simulink model "pfb_core_snbxfft32"  (R2012b)
settings: Solver=FixedStepDiscrete  SolverMode=SingleTasking  StartTime=0.0  StopTime=5000  FixedStep=1  RelTol=1e-3
undefined symbols (not defined in the file or in its folder): xlipgetpartsetting
undefined symbols (not defined in the file): pfb_coeff_gen_calc
libraries: xbsIndex_r4 x5100, casper_library_misc x2, casper_library_delays x1
(part 4 of 18)

== system pfb_core_snbxfft32/pfb/pfb_fir_generic/pfb_fir_coeff_gen/rom ==
  addra : Inport
  dina : Inport  Port=2
  wea : Inport  Port=3
  addrb : Inport  Port=4
  dinb : Inport  Port=5
  web : Inport  Port=6
  A_bussify : Subsystem  AncestorBlock=casper_library_flow_control/bus_create  mask(bus_create){inputNum=72}
      mask prompts: inputNum "Number of inputs:"
      mask init:
      | bus_create_init(gcb,...
      |     'inputNum', inputNum);
  B_bussify : Subsystem  AncestorBlock=casper_library_flow_control/bus_create  mask(bus_create){inputNum=72}
      mask prompts: inputNum "Number of inputs:"
      mask init:
      | bus_create_init(gcb,...
      |     'inputNum', inputNum);
  bram{0..71} (72 alike) : xbsIndex_r4/Dual Port RAM  depth=65536  initVector=getfield(get_param(gcb, 'UserData'), 'initVector')  distributed_mem=Block RAM  init_a=0  init_b=0  rst_a=off  rst_b=off  en_a=off  en_b=off  latency=8  write_mode_A=Read Before Write  write_mode_B=Read Before Write  dbl_ovrd=off  optimize=Speed  block_type=dpram
  ddina : xbsIndex_r4/Delay  rst=off  infoeditControl=Selection of Reset will increase slice count due to use of real FFs and instead of SRLs  en=off  latency=0  dbl_ovrd=off  reg_retiming=on  block_type=delay
  ddinb : xbsIndex_r4/Delay  rst=off  infoeditControl=Selection of Reset will increase slice count due to use of real FFs and instead of SRLs  en=off  latency=0  dbl_ovrd=off  reg_retiming=on  block_type=delay
  debus_addra : Subsystem  AncestorBlock=casper_library_flow_control/bus_expand  mask(bus_expand){mode=divisions of equal size, outputNum=72, outputWidth=[16 16 16 16 16 16 16 16 16 16 16 16 16 16 16 16 16 16 16 16 16 16 16 16 16 16 16 16 16 16 16 16 16 16 16 16 16 16 16 16 16 16 16 16 16 16 16 16 16 16 16 16 16 16 16 16 16 16 16 16 16 16 16 16 16 16 16 16 16 16 16 16], outputBinaryPt=[0 0 0 0 0 0 0 0 0 0 0 0 0 0 0 0 0 0 0 0 0 0 0 0 0 0 0 0 0 0 0 0 0 0 0 0 0 0 0 0 0 0 0 0 0 0 0 0 0 0 0 0 0 0 0 0 0 0 0 0 0 0 0 0 0 0 0 0 0 0 0 0], outputArithmeticType=[0 0 0 0 0 0 0 0 0 0 0 0 0 0 0 0 0 0 0 0 0 0 0 0 0 0 0 0 0 0 0 0 0 0 0 0 0 0 0 0 0 0 0 0 0 0 0 0 0 0 0 0 0 0 0 0 0 0 0 0 0 0 0 0 0 0 0 0 0 0 0 0], show_format=on, outputToWorkspace=off, variablePrefix=, outputToModelAsWell=on}
      mask prompts: outputNum "Number of outputs:"; outputWidth "Output width:"; outputBinaryPt "Output binary point position:"; outputArithmeticType "Output arithmetic type (ufix=0, fix=1, bool=2):"; show_format "Print format string?"; outputToWorkspace "Output to workspace?"; variablePrefix "Variable name prefix:"; outputToModelAsWell "Output to model as well?"
      mask help:
      | Expands a 'bus' made using a bus_create or Xilinx
      | concat block.
      | The input will be divided into the specified number
      | of outputs with the specified arithmetic types.
      | Divisions are made from most significant bit.
      mask init: same as pfb_core_snbxfft32/pfb/pfb_fir_generic/bus_expand
      settings: AttributesFormatString=72 outputs: uf16.0,uf16.0,uf16.0,uf16.0,uf16.0,uf16.0,uf16.0,uf16.0,uf16.0,uf16.0,uf16.0,uf16.0,uf16.0,uf16.0,uf16.0,uf16.0,uf16.0,uf16.0,uf16.0,uf16.0,uf16.0,uf16.0,uf16.0,uf16.0,uf16.0,uf16.0,uf16.0,uf16.0,uf16.0,uf16.0,uf16.0,uf16.0,uf16.0,uf16.0,uf16.0,uf16.0,uf16.0,uf16.0,uf16.0,uf16.0,uf16.0,uf16.0,uf16.0,uf16.0,uf16.0,uf16.0,uf16.0,uf16.0,uf16.0,uf16.0,uf16.0,uf16.0,uf16.0,uf16.0,uf16.0,uf16.0,uf16.0,uf16.0,uf16.0,uf16.0,uf16.0,uf16.0,uf16.0,uf16.0,uf16.0,uf16.0,uf16.0,uf16.0,uf16.0,uf16.0,uf16.0,uf16.0,
      mask TypeOptions mode: divisions of equal size | divisions of arbitrary size
      mask Callback mode: bus_expand_callback();
      mask Callback outputWidth: bus_expand_callback();
      mask Callback outputToWorkspace: bus_expand_callback();
  debus_addrb : Subsystem  AncestorBlock=casper_library_flow_control/bus_expand  mask(bus_expand){mode=divisions of equal size, outputNum=72, outputWidth=[16 16 16 16 16 16 16 16 16 16 16 16 16 16 16 16 16 16 16 16 16 16 16 16 16 16 16 16 16 16 16 16 16 16 16 16 16 16 16 16 16 16 16 16 16 16 16 16 16 16 16 16 16 16 16 16 16 16 16 16 16 16 16 16 16 16 16 16 16 16 16 16], outputBinaryPt=[0 0 0 0 0 0 0 0 0 0 0 0 0 0 0 0 0 0 0 0 0 0 0 0 0 0 0 0 0 0 0 0 0 0 0 0 0 0 0 0 0 0 0 0 0 0 0 0 0 0 0 0 0 0 0 0 0 0 0 0 0 0 0 0 0 0 0 0 0 0 0 0], outputArithmeticType=[0 0 0 0 0 0 0 0 0 0 0 0 0 0 0 0 0 0 0 0 0 0 0 0 0 0 0 0 0 0 0 0 0 0 0 0 0 0 0 0 0 0 0 0 0 0 0 0 0 0 0 0 0 0 0 0 0 0 0 0 0 0 0 0 0 0 0 0 0 0 0 0], show_format=on, outputToWorkspace=off, variablePrefix=, outputToModelAsWell=on}
      mask prompts: outputNum "Number of outputs:"; outputWidth "Output width:"; outputBinaryPt "Output binary point position:"; outputArithmeticType "Output arithmetic type (ufix=0, fix=1, bool=2):"; show_format "Print format string?"; outputToWorkspace "Output to workspace?"; variablePrefix "Variable name prefix:"; outputToModelAsWell "Output to model as well?"
      mask help:
      | Expands a 'bus' made using a bus_create or Xilinx
      | concat block.
      | The input will be divided into the specified number
      | of outputs with the specified arithmetic types.
      | Divisions are made from most significant bit.
      mask init: same as pfb_core_snbxfft32/pfb/pfb_fir_generic/bus_expand
      settings: AttributesFormatString=72 outputs: uf16.0,uf16.0,uf16.0,uf16.0,uf16.0,uf16.0,uf16.0,uf16.0,uf16.0,uf16.0,uf16.0,uf16.0,uf16.0,uf16.0,uf16.0,uf16.0,uf16.0,uf16.0,uf16.0,uf16.0,uf16.0,uf16.0,uf16.0,uf16.0,uf16.0,uf16.0,uf16.0,uf16.0,uf16.0,uf16.0,uf16.0,uf16.0,uf16.0,uf16.0,uf16.0,uf16.0,uf16.0,uf16.0,uf16.0,uf16.0,uf16.0,uf16.0,uf16.0,uf16.0,uf16.0,uf16.0,uf16.0,uf16.0,uf16.0,uf16.0,uf16.0,uf16.0,uf16.0,uf16.0,uf16.0,uf16.0,uf16.0,uf16.0,uf16.0,uf16.0,uf16.0,uf16.0,uf16.0,uf16.0,uf16.0,uf16.0,uf16.0,uf16.0,uf16.0,uf16.0,uf16.0,uf16.0,
      mask TypeOptions mode: divisions of equal size | divisions of arbitrary size
      mask Callback mode: bus_expand_callback();
      mask Callback outputWidth: bus_expand_callback();
      mask Callback outputToWorkspace: bus_expand_callback();
  debus_dina : Subsystem  AncestorBlock=casper_library_flow_control/bus_expand  mask(bus_expand){mode=divisions of arbitrary size, outputNum=1, outputWidth=[1 1 1 1 1 1 1 1 1 1 1 1 1 1 1 1 1 1 1 1 1 1 1 1 1 1 1 1 1 1 1 1 1 1 1 1 1 1 1 1 1 1 1 1 1 1 1 1 1 1 1 1 1 1 1 1 1 1 1 1 1 1 1 1 1 1 1 1 1 1 1 1], outputBinaryPt=[0 0 0 0 0 0 0 0 0 0 0 0 0 0 0 0 0 0 0 0 0 0 0 0 0 0 0 0 0 0 0 0 0 0 0 0 0 0 0 0 0 0 0 0 0 0 0 0 0 0 0 0 0 0 0 0 0 0 0 0 0 0 0 0 0 0 0 0 0 0 0 0], outputArithmeticType=[0 0 0 0 0 0 0 0 0 0 0 0 0 0 0 0 0 0 0 0 0 0 0 0 0 0 0 0 0 0 0 0 0 0 0 0 0 0 0 0 0 0 0 0 0 0 0 0 0 0 0 0 0 0 0 0 0 0 0 0 0 0 0 0 0 0 0 0 0 0 0 0], show_format=on, outputToWorkspace=off, variablePrefix=, outputToModelAsWell=on}
      mask prompts: outputNum "Number of outputs:"; outputWidth "Output width [msb ... lsb]:"; outputBinaryPt "Output binary point position [msb ... lsb]:"; outputArithmeticType "Output arithmetic type (ufix=0, fix=1, bool=2) [msb ... lsb]:"; show_format "Print format string?"; outputToWorkspace "Output to workspace?"; variablePrefix "Variable name prefix:"; outputToModelAsWell "Output to model as well?"
      mask help:
      | Expands a 'bus' made using a bus_create or Xilinx
      | concat block.
      | The input will be divided into the specified number
      | of outputs with the specified arithmetic types.
      | Divisions are made from most significant bit.
      mask init: same as pfb_core_snbxfft32/pfb/pfb_fir_generic/bus_expand
      settings: AttributesFormatString=72 outputs: uf1.0,uf1.0,uf1.0,uf1.0,uf1.0,uf1.0,uf1.0,uf1.0,uf1.0,uf1.0,uf1.0,uf1.0,uf1.0,uf1.0,uf1.0,uf1.0,uf1.0,uf1.0,uf1.0,uf1.0,uf1.0,uf1.0,uf1.0,uf1.0,uf1.0,uf1.0,uf1.0,uf1.0,uf1.0,uf1.0,uf1.0,uf1.0,uf1.0,uf1.0,uf1.0,uf1.0,uf1.0,uf1.0,uf1.0,uf1.0,uf1.0,uf1.0,uf1.0,uf1.0,uf1.0,uf1.0,uf1.0,uf1.0,uf1.0,uf1.0,uf1.0,uf1.0,uf1.0,uf1.0,uf1.0,uf1.0,uf1.0,uf1.0,uf1.0,uf1.0,uf1.0,uf1.0,uf1.0,uf1.0,uf1.0,uf1.0,uf1.0,uf1.0,uf1.0,uf1.0,uf1.0,uf1.0,
      mask TypeOptions mode: divisions of equal size | divisions of arbitrary size
      mask Callback mode: bus_expand_callback();
      mask Callback outputWidth: bus_expand_callback();
      mask Callback outputToWorkspace: bus_expand_callback();
  debus_dinb : Subsystem  AncestorBlock=casper_library_flow_control/bus_expand  mask(bus_expand){mode=divisions of arbitrary size, outputNum=1, outputWidth=[1 1 1 1 1 1 1 1 1 1 1 1 1 1 1 1 1 1 1 1 1 1 1 1 1 1 1 1 1 1 1 1 1 1 1 1 1 1 1 1 1 1 1 1 1 1 1 1 1 1 1 1 1 1 1 1 1 1 1 1 1 1 1 1 1 1 1 1 1 1 1 1], outputBinaryPt=[0 0 0 0 0 0 0 0 0 0 0 0 0 0 0 0 0 0 0 0 0 0 0 0 0 0 0 0 0 0 0 0 0 0 0 0 0 0 0 0 0 0 0 0 0 0 0 0 0 0 0 0 0 0 0 0 0 0 0 0 0 0 0 0 0 0 0 0 0 0 0 0], outputArithmeticType=[0 0 0 0 0 0 0 0 0 0 0 0 0 0 0 0 0 0 0 0 0 0 0 0 0 0 0 0 0 0 0 0 0 0 0 0 0 0 0 0 0 0 0 0 0 0 0 0 0 0 0 0 0 0 0 0 0 0 0 0 0 0 0 0 0 0 0 0 0 0 0 0], show_format=on, outputToWorkspace=off, variablePrefix=, outputToModelAsWell=on}
      mask prompts: outputNum "Number of outputs:"; outputWidth "Output width [msb ... lsb]:"; outputBinaryPt "Output binary point position [msb ... lsb]:"; outputArithmeticType "Output arithmetic type (ufix=0, fix=1, bool=2) [msb ... lsb]:"; show_format "Print format string?"; outputToWorkspace "Output to workspace?"; variablePrefix "Variable name prefix:"; outputToModelAsWell "Output to model as well?"
      mask help:
      | Expands a 'bus' made using a bus_create or Xilinx
      | concat block.
      | The input will be divided into the specified number
      | of outputs with the specified arithmetic types.
      | Divisions are made from most significant bit.
      mask init: same as pfb_core_snbxfft32/pfb/pfb_fir_generic/bus_expand
      settings: AttributesFormatString=72 outputs: uf1.0,uf1.0,uf1.0,uf1.0,uf1.0,uf1.0,uf1.0,uf1.0,uf1.0,uf1.0,uf1.0,uf1.0,uf1.0,uf1.0,uf1.0,uf1.0,uf1.0,uf1.0,uf1.0,uf1.0,uf1.0,uf1.0,uf1.0,uf1.0,uf1.0,uf1.0,uf1.0,uf1.0,uf1.0,uf1.0,uf1.0,uf1.0,uf1.0,uf1.0,uf1.0,uf1.0,uf1.0,uf1.0,uf1.0,uf1.0,uf1.0,uf1.0,uf1.0,uf1.0,uf1.0,uf1.0,uf1.0,uf1.0,uf1.0,uf1.0,uf1.0,uf1.0,uf1.0,uf1.0,uf1.0,uf1.0,uf1.0,uf1.0,uf1.0,uf1.0,uf1.0,uf1.0,uf1.0,uf1.0,uf1.0,uf1.0,uf1.0,uf1.0,uf1.0,uf1.0,uf1.0,uf1.0,
      mask TypeOptions mode: divisions of equal size | divisions of arbitrary size
      mask Callback mode: bus_expand_callback();
      mask Callback outputWidth: bus_expand_callback();
      mask Callback outputToWorkspace: bus_expand_callback();
  debus_wea : Subsystem  AncestorBlock=casper_library_flow_control/bus_expand  mask(bus_expand){mode=divisions of equal size, outputNum=72, outputWidth=[1 1 1 1 1 1 1 1 1 1 1 1 1 1 1 1 1 1 1 1 1 1 1 1 1 1 1 1 1 1 1 1 1 1 1 1 1 1 1 1 1 1 1 1 1 1 1 1 1 1 1 1 1 1 1 1 1 1 1 1 1 1 1 1 1 1 1 1 1 1 1 1], outputBinaryPt=[0 0 0 0 0 0 0 0 0 0 0 0 0 0 0 0 0 0 0 0 0 0 0 0 0 0 0 0 0 0 0 0 0 0 0 0 0 0 0 0 0 0 0 0 0 0 0 0 0 0 0 0 0 0 0 0 0 0 0 0 0 0 0 0 0 0 0 0 0 0 0 0], outputArithmeticType=[2 2 2 2 2 2 2 2 2 2 2 2 2 2 2 2 2 2 2 2 2 2 2 2 2 2 2 2 2 2 2 2 2 2 2 2 2 2 2 2 2 2 2 2 2 2 2 2 2 2 2 2 2 2 2 2 2 2 2 2 2 2 2 2 2 2 2 2 2 2 2 2], show_format=on, outputToWorkspace=off, variablePrefix=, outputToModelAsWell=on}
      mask prompts: outputNum "Number of outputs:"; outputWidth "Output width:"; outputBinaryPt "Output binary point position:"; outputArithmeticType "Output arithmetic type (ufix=0, fix=1, bool=2):"; show_format "Print format string?"; outputToWorkspace "Output to workspace?"; variablePrefix "Variable name prefix:"; outputToModelAsWell "Output to model as well?"
      mask help:
      | Expands a 'bus' made using a bus_create or Xilinx
      | concat block.
      | The input will be divided into the specified number
      | of outputs with the specified arithmetic types.
      | Divisions are made from most significant bit.
      mask init: same as pfb_core_snbxfft32/pfb/pfb_fir_generic/bus_expand
      settings: AttributesFormatString=72 outputs: b,b,b,b,b,b,b,b,b,b,b,b,b,b,b,b,b,b,b,b,b,b,b,b,b,b,b,b,b,b,b,b,b,b,b,b,b,b,b,b,b,b,b,b,b,b,b,b,b,b,b,b,b,b,b,b,b,b,b,b,b,b,b,b,b,b,b,b,b,b,b,b,
      mask TypeOptions mode: divisions of equal size | divisions of arbitrary size
      mask Callback mode: bus_expand_callback();
      mask Callback outputWidth: bus_expand_callback();
      mask Callback outputToWorkspace: bus_expand_callback();
  debus_web : Subsystem  AncestorBlock=casper_library_flow_control/bus_expand  mask(bus_expand){mode=divisions of equal size, outputNum=72, outputWidth=[1 1 1 1 1 1 1 1 1 1 1 1 1 1 1 1 1 1 1 1 1 1 1 1 1 1 1 1 1 1 1 1 1 1 1 1 1 1 1 1 1 1 1 1 1 1 1 1 1 1 1 1 1 1 1 1 1 1 1 1 1 1 1 1 1 1 1 1 1 1 1 1], outputBinaryPt=[0 0 0 0 0 0 0 0 0 0 0 0 0 0 0 0 0 0 0 0 0 0 0 0 0 0 0 0 0 0 0 0 0 0 0 0 0 0 0 0 0 0 0 0 0 0 0 0 0 0 0 0 0 0 0 0 0 0 0 0 0 0 0 0 0 0 0 0 0 0 0 0], outputArithmeticType=[2 2 2 2 2 2 2 2 2 2 2 2 2 2 2 2 2 2 2 2 2 2 2 2 2 2 2 2 2 2 2 2 2 2 2 2 2 2 2 2 2 2 2 2 2 2 2 2 2 2 2 2 2 2 2 2 2 2 2 2 2 2 2 2 2 2 2 2 2 2 2 2], show_format=on, outputToWorkspace=off, variablePrefix=, outputToModelAsWell=on}
      mask prompts: outputNum "Number of outputs:"; outputWidth "Output width:"; outputBinaryPt "Output binary point position:"; outputArithmeticType "Output arithmetic type (ufix=0, fix=1, bool=2):"; show_format "Print format string?"; outputToWorkspace "Output to workspace?"; variablePrefix "Variable name prefix:"; outputToModelAsWell "Output to model as well?"
      mask help:
      | Expands a 'bus' made using a bus_create or Xilinx
      | concat block.
      | The input will be divided into the specified number
      | of outputs with the specified arithmetic types.
      | Divisions are made from most significant bit.
      mask init: same as pfb_core_snbxfft32/pfb/pfb_fir_generic/bus_expand
      settings: AttributesFormatString=72 outputs: b,b,b,b,b,b,b,b,b,b,b,b,b,b,b,b,b,b,b,b,b,b,b,b,b,b,b,b,b,b,b,b,b,b,b,b,b,b,b,b,b,b,b,b,b,b,b,b,b,b,b,b,b,b,b,b,b,b,b,b,b,b,b,b,b,b,b,b,b,b,b,b,
      mask TypeOptions mode: divisions of equal size | divisions of arbitrary size
      mask Callback mode: bus_expand_callback();
      mask Callback outputWidth: bus_expand_callback();
      mask Callback outputToWorkspace: bus_expand_callback();
  rep_addra : Subsystem  AncestorBlock=casper_library_bus/bus_replicate  mask(bus_replicate){replication=72, latency=9, misc=off, implementation=core}
      mask prompts: replication "replication factor"; misc "misc support"; implementation "delay implementation"
      mask help: Output bus formed by replicating input bus a number of times
      mask init:
      | bus_replicate_init(gcb, ...
      |     'replication', replication, ...
      |     'latency', latency, ...
      |     'implementation', implementation, ...
      |     'misc', misc);
      mask TypeOptions implementation: core | behavioral
  rep_addrb : Subsystem  AncestorBlock=casper_library_bus/bus_replicate  mask(bus_replicate){replication=72, latency=9, misc=off, implementation=core}
      mask prompts: replication "replication factor"; misc "misc support"; implementation "delay implementation"
      mask help: Output bus formed by replicating input bus a number of times
      mask init:
      | bus_replicate_init(gcb, ...
      |     'replication', replication, ...
      |     'latency', latency, ...
      |     'implementation', implementation, ...
      |     'misc', misc);
      mask TypeOptions implementation: core | behavioral
  rep_wea : Subsystem  AncestorBlock=casper_library_bus/bus_replicate  mask(bus_replicate){replication=72, latency=0, misc=off, implementation=behavioral}
      mask prompts: replication "replication factor"; misc "misc support"; implementation "delay implementation"
      mask help: Output bus formed by replicating input bus a number of times
      mask init:
      | bus_replicate_init(gcb, ...
      |     'replication', replication, ...
      |     'latency', latency, ...
      |     'implementation', implementation, ...
      |     'misc', misc);
      mask TypeOptions implementation: core | behavioral
  rep_web : Subsystem  AncestorBlock=casper_library_bus/bus_replicate  mask(bus_replicate){replication=72, latency=0, misc=off, implementation=behavioral}
      mask prompts: replication "replication factor"; misc "misc support"; implementation "delay implementation"
      mask help: Output bus formed by replicating input bus a number of times
      mask init:
      | bus_replicate_init(gcb, ...
      |     'replication', replication, ...
      |     'latency', latency, ...
      |     'implementation', implementation, ...
      |     'misc', misc);
      mask TypeOptions implementation: core | behavioral
  A : Outport
  B : Outport  Port=2
  wires:
  addra/1 -> rep_addra/1(in)
  dina/1 -> ddina/1
  wea/1 -> rep_wea/1(in)
  addrb/1 -> rep_addrb/1(in)
  dinb/1 -> ddinb/1
  web/1 -> rep_web/1(in)
  rep_addra/1(out) -> debus_addra/1(bus_in)
  ddina/1 -> debus_dina/1(bus_in)
  rep_wea/1(out) -> debus_wea/1(bus_in)
  rep_addrb/1(out) -> debus_addrb/1(bus_in)
  ddinb/1 -> debus_dinb/1(bus_in)
  rep_web/1(out) -> debus_web/1(bus_in)
  debus_addra/1(msb_out72) -> bram0/1
  debus_dina/1(msb_out72) -> bram0/2
  debus_wea/1(msb_out72) -> bram0/3
  debus_addrb/1(msb_out72) -> bram0/4
  debus_dinb/1(msb_out72) -> bram0/5
  debus_web/1(msb_out72) -> bram0/6
  debus_addra/2(out71) -> bram1/1
  debus_dina/2(out71) -> bram1/2
  debus_wea/2(out71) -> bram1/3
  debus_addrb/2(out71) -> bram1/4
  debus_dinb/2(out71) -> bram1/5
  debus_web/2(out71) -> bram1/6
  debus_addra/3(out70) -> bram2/1
  debus_dina/3(out70) -> bram2/2
  debus_wea/3(out70) -> bram2/3
  debus_addrb/3(out70) -> bram2/4
  debus_dinb/3(out70) -> bram2/5
  debus_web/3(out70) -> bram2/6
  debus_addra/4(out69) -> bram3/1
  debus_dina/4(out69) -> bram3/2
  debus_wea/4(out69) -> bram3/3
  debus_addrb/4(out69) -> bram3/4
  debus_dinb/4(out69) -> bram3/5
  debus_web/4(out69) -> bram3/6
  debus_addra/5(out68) -> bram4/1
  debus_dina/5(out68) -> bram4/2
  debus_wea/5(out68) -> bram4/3
  debus_addrb/5(out68) -> bram4/4
  debus_dinb/5(out68) -> bram4/5
  debus_web/5(out68) -> bram4/6
  debus_addra/6(out67) -> bram5/1
  debus_dina/6(out67) -> bram5/2
  debus_wea/6(out67) -> bram5/3
  debus_addrb/6(out67) -> bram5/4
  debus_dinb/6(out67) -> bram5/5
  debus_web/6(out67) -> bram5/6
  debus_addra/7(out66) -> bram6/1
  debus_dina/7(out66) -> bram6/2
  debus_wea/7(out66) -> bram6/3
  debus_addrb/7(out66) -> bram6/4
  debus_dinb/7(out66) -> bram6/5
  debus_web/7(out66) -> bram6/6
  debus_addra/8(out65) -> bram7/1
  debus_dina/8(out65) -> bram7/2
  debus_wea/8(out65) -> bram7/3
  debus_addrb/8(out65) -> bram7/4
  debus_dinb/8(out65) -> bram7/5
  debus_web/8(out65) -> bram7/6
  debus_addra/9(out64) -> bram8/1
  debus_dina/9(out64) -> bram8/2
  debus_wea/9(out64) -> bram8/3
  debus_addrb/9(out64) -> bram8/4
  debus_dinb/9(out64) -> bram8/5
  debus_web/9(out64) -> bram8/6
  debus_addra/10(out63) -> bram9/1
  debus_dina/10(out63) -> bram9/2
  debus_wea/10(out63) -> bram9/3
  debus_addrb/10(out63) -> bram9/4
  debus_dinb/10(out63) -> bram9/5
  debus_web/10(out63) -> bram9/6
  debus_addra/11(out62) -> bram10/1
  debus_dina/11(out62) -> bram10/2
  debus_wea/11(out62) -> bram10/3
  debus_addrb/11(out62) -> bram10/4
  debus_dinb/11(out62) -> bram10/5
  debus_web/11(out62) -> bram10/6
  debus_addra/12(out61) -> bram11/1
  debus_dina/12(out61) -> bram11/2
  debus_wea/12(out61) -> bram11/3
  debus_addrb/12(out61) -> bram11/4
  debus_dinb/12(out61) -> bram11/5
  debus_web/12(out61) -> bram11/6
  debus_addra/13(out60) -> bram12/1
  debus_dina/13(out60) -> bram12/2
  debus_wea/13(out60) -> bram12/3
  debus_addrb/13(out60) -> bram12/4
  debus_dinb/13(out60) -> bram12/5
  debus_web/13(out60) -> bram12/6
  debus_addra/14(out59) -> bram13/1
  debus_dina/14(out59) -> bram13/2
  debus_wea/14(out59) -> bram13/3
  debus_addrb/14(out59) -> bram13/4
  debus_dinb/14(out59) -> bram13/5
  debus_web/14(out59) -> bram13/6
  debus_addra/15(out58) -> bram14/1
  debus_dina/15(out58) -> bram14/2
  debus_wea/15(out58) -> bram14/3
  debus_addrb/15(out58) -> bram14/4
  debus_dinb/15(out58) -> bram14/5
  debus_web/15(out58) -> bram14/6
  debus_addra/16(out57) -> bram15/1
  debus_dina/16(out57) -> bram15/2
  debus_wea/16(out57) -> bram15/3
  debus_addrb/16(out57) -> bram15/4
  debus_dinb/16(out57) -> bram15/5
  debus_web/16(out57) -> bram15/6
  debus_addra/17(out56) -> bram16/1
  debus_dina/17(out56) -> bram16/2
  debus_wea/17(out56) -> bram16/3
  debus_addrb/17(out56) -> bram16/4
  debus_dinb/17(out56) -> bram16/5
  debus_web/17(out56) -> bram16/6
  debus_addra/18(out55) -> bram17/1
  debus_dina/18(out55) -> bram17/2
  debus_wea/18(out55) -> bram17/3
  debus_addrb/18(out55) -> bram17/4
  debus_dinb/18(out55) -> bram17/5
  debus_web/18(out55) -> bram17/6
  debus_addra/19(out54) -> bram18/1
  debus_dina/19(out54) -> bram18/2
  debus_wea/19(out54) -> bram18/3
  debus_addrb/19(out54) -> bram18/4
  debus_dinb/19(out54) -> bram18/5
  debus_web/19(out54) -> bram18/6
  debus_addra/20(out53) -> bram19/1
  debus_dina/20(out53) -> bram19/2
  debus_wea/20(out53) -> bram19/3
  debus_addrb/20(out53) -> bram19/4
  debus_dinb/20(out53) -> bram19/5
  debus_web/20(out53) -> bram19/6
  debus_addra/21(out52) -> bram20/1
  debus_dina/21(out52) -> bram20/2
  debus_wea/21(out52) -> bram20/3
  debus_addrb/21(out52) -> bram20/4
  debus_dinb/21(out52) -> bram20/5
  debus_web/21(out52) -> bram20/6
  debus_addra/22(out51) -> bram21/1
  debus_dina/22(out51) -> bram21/2
  debus_wea/22(out51) -> bram21/3
  debus_addrb/22(out51) -> bram21/4
  debus_dinb/22(out51) -> bram21/5
  debus_web/22(out51) -> bram21/6
  debus_addra/23(out50) -> bram22/1
  debus_dina/23(out50) -> bram22/2
  debus_wea/23(out50) -> bram22/3
  debus_addrb/23(out50) -> bram22/4
  debus_dinb/23(out50) -> bram22/5
  debus_web/23(out50) -> bram22/6
  debus_addra/24(out49) -> bram23/1
  debus_dina/24(out49) -> bram23/2
  debus_wea/24(out49) -> bram23/3
  debus_addrb/24(out49) -> bram23/4
  debus_dinb/24(out49) -> bram23/5
  debus_web/24(out49) -> bram23/6
  debus_addra/25(out48) -> bram24/1
  debus_dina/25(out48) -> bram24/2
  debus_wea/25(out48) -> bram24/3
  debus_addrb/25(out48) -> bram24/4
  debus_dinb/25(out48) -> bram24/5
  debus_web/25(out48) -> bram24/6
  debus_addra/26(out47) -> bram25/1
  debus_dina/26(out47) -> bram25/2
  debus_wea/26(out47) -> bram25/3
  debus_addrb/26(out47) -> bram25/4
  debus_dinb/26(out47) -> bram25/5
  debus_web/26(out47) -> bram25/6
  debus_addra/27(out46) -> bram26/1
  debus_dina/27(out46) -> bram26/2
  debus_wea/27(out46) -> bram26/3
  debus_addrb/27(out46) -> bram26/4
  debus_dinb/27(out46) -> bram26/5
  debus_web/27(out46) -> bram26/6
  debus_addra/28(out45) -> bram27/1
  debus_dina/28(out45) -> bram27/2
  debus_wea/28(out45) -> bram27/3
  debus_addrb/28(out45) -> bram27/4
  debus_dinb/28(out45) -> bram27/5
  debus_web/28(out45) -> bram27/6
  debus_addra/29(out44) -> bram28/1
  debus_dina/29(out44) -> bram28/2
  debus_wea/29(out44) -> bram28/3
  debus_addrb/29(out44) -> bram28/4
  debus_dinb/29(out44) -> bram28/5
  debus_web/29(out44) -> bram28/6
  debus_addra/30(out43) -> bram29/1
  debus_dina/30(out43) -> bram29/2
  debus_wea/30(out43) -> bram29/3
  debus_addrb/30(out43) -> bram29/4
  debus_dinb/30(out43) -> bram29/5
  debus_web/30(out43) -> bram29/6
  debus_addra/31(out42) -> bram30/1
  debus_dina/31(out42) -> bram30/2
  debus_wea/31(out42) -> bram30/3
  debus_addrb/31(out42) -> bram30/4
  debus_dinb/31(out42) -> bram30/5
  debus_web/31(out42) -> bram30/6
  debus_addra/32(out41) -> bram31/1
  debus_dina/32(out41) -> bram31/2
  debus_wea/32(out41) -> bram31/3
  debus_addrb/32(out41) -> bram31/4
  debus_dinb/32(out41) -> bram31/5
  debus_web/32(out41) -> bram31/6
  debus_addra/33(out40) -> bram32/1
  debus_dina/33(out40) -> bram32/2
  debus_wea/33(out40) -> bram32/3
  debus_addrb/33(out40) -> bram32/4
  debus_dinb/33(out40) -> bram32/5
  debus_web/33(out40) -> bram32/6
  debus_addra/34(out39) -> bram33/1
  debus_dina/34(out39) -> bram33/2
  debus_wea/34(out39) -> bram33/3
  debus_addrb/34(out39) -> bram33/4
  debus_dinb/34(out39) -> bram33/5
  debus_web/34(out39) -> bram33/6
  debus_addra/35(out38) -> bram34/1
  debus_dina/35(out38) -> bram34/2
  debus_wea/35(out38) -> bram34/3
  debus_addrb/35(out38) -> bram34/4
  debus_dinb/35(out38) -> bram34/5
  debus_web/35(out38) -> bram34/6
  debus_addra/36(out37) -> bram35/1
  debus_dina/36(out37) -> bram35/2
  debus_wea/36(out37) -> bram35/3
  debus_addrb/36(out37) -> bram35/4
  debus_dinb/36(out37) -> bram35/5
  debus_web/36(out37) -> bram35/6
  debus_addra/37(out36) -> bram36/1
  debus_dina/37(out36) -> bram36/2
  debus_wea/37(out36) -> bram36/3
  debus_addrb/37(out36) -> bram36/4
  debus_dinb/37(out36) -> bram36/5
  debus_web/37(out36) -> bram36/6
  debus_addra/38(out35) -> bram37/1
  debus_dina/38(out35) -> bram37/2
  debus_wea/38(out35) -> bram37/3
  debus_addrb/38(out35) -> bram37/4
  debus_dinb/38(out35) -> bram37/5
  debus_web/38(out35) -> bram37/6
  debus_addra/39(out34) -> bram38/1
  debus_dina/39(out34) -> bram38/2
  debus_wea/39(out34) -> bram38/3
  debus_addrb/39(out34) -> bram38/4
  debus_dinb/39(out34) -> bram38/5
  debus_web/39(out34) -> bram38/6
  debus_addra/40(out33) -> bram39/1
  debus_dina/40(out33) -> bram39/2
  debus_wea/40(out33) -> bram39/3
  debus_addrb/40(out33) -> bram39/4
  debus_dinb/40(out33) -> bram39/5
  debus_web/40(out33) -> bram39/6
  debus_addra/41(out32) -> bram40/1
  debus_dina/41(out32) -> bram40/2
  debus_wea/41(out32) -> bram40/3
  debus_addrb/41(out32) -> bram40/4
  debus_dinb/41(out32) -> bram40/5
  debus_web/41(out32) -> bram40/6
  debus_addra/42(out31) -> bram41/1
  debus_dina/42(out31) -> bram41/2
  debus_wea/42(out31) -> bram41/3
  debus_addrb/42(out31) -> bram41/4
  debus_dinb/42(out31) -> bram41/5
  debus_web/42(out31) -> bram41/6
  debus_addra/43(out30) -> bram42/1
  debus_dina/43(out30) -> bram42/2
  debus_wea/43(out30) -> bram42/3
  debus_addrb/43(out30) -> bram42/4
  debus_dinb/43(out30) -> bram42/5
  debus_web/43(out30) -> bram42/6
  debus_addra/44(out29) -> bram43/1
  debus_dina/44(out29) -> bram43/2
  debus_wea/44(out29) -> bram43/3
  debus_addrb/44(out29) -> bram43/4
  debus_dinb/44(out29) -> bram43/5
  debus_web/44(out29) -> bram43/6
  debus_addra/45(out28) -> bram44/1
  debus_dina/45(out28) -> bram44/2
  debus_wea/45(out28) -> bram44/3
  debus_addrb/45(out28) -> bram44/4
  debus_dinb/45(out28) -> bram44/5
  debus_web/45(out28) -> bram44/6
  debus_addra/46(out27) -> bram45/1
  debus_dina/46(out27) -> bram45/2
  debus_wea/46(out27) -> bram45/3
  debus_addrb/46(out27) -> bram45/4
  debus_dinb/46(out27) -> bram45/5
  debus_web/46(out27) -> bram45/6
  debus_addra/47(out26) -> bram46/1
  debus_dina/47(out26) -> bram46/2
  debus_wea/47(out26) -> bram46/3
  debus_addrb/47(out26) -> bram46/4
  debus_dinb/47(out26) -> bram46/5
  debus_web/47(out26) -> bram46/6
  debus_addra/48(out25) -> bram47/1
  debus_dina/48(out25) -> bram47/2
  debus_wea/48(out25) -> bram47/3
  debus_addrb/48(out25) -> bram47/4
  debus_dinb/48(out25) -> bram47/5
  debus_web/48(out25) -> bram47/6
  debus_addra/49(out24) -> bram48/1
  debus_dina/49(out24) -> bram48/2
  debus_wea/49(out24) -> bram48/3
  debus_addrb/49(out24) -> bram48/4
  debus_dinb/49(out24) -> bram48/5
  debus_web/49(out24) -> bram48/6
  debus_addra/50(out23) -> bram49/1
  debus_dina/50(out23) -> bram49/2
  debus_wea/50(out23) -> bram49/3
  debus_addrb/50(out23) -> bram49/4
  debus_dinb/50(out23) -> bram49/5
  debus_web/50(out23) -> bram49/6
  debus_addra/51(out22) -> bram50/1
  debus_dina/51(out22) -> bram50/2
  debus_wea/51(out22) -> bram50/3
  debus_addrb/51(out22) -> bram50/4
  debus_dinb/51(out22) -> bram50/5
  debus_web/51(out22) -> bram50/6
  debus_addra/52(out21) -> bram51/1
  debus_dina/52(out21) -> bram51/2
  debus_wea/52(out21) -> bram51/3
  debus_addrb/52(out21) -> bram51/4
  debus_dinb/52(out21) -> bram51/5
  debus_web/52(out21) -> bram51/6
  debus_addra/53(out20) -> bram52/1
  debus_dina/53(out20) -> bram52/2
  debus_wea/53(out20) -> bram52/3
  debus_addrb/53(out20) -> bram52/4
  debus_dinb/53(out20) -> bram52/5
  debus_web/53(out20) -> bram52/6
  debus_addra/54(out19) -> bram53/1
  debus_dina/54(out19) -> bram53/2
  debus_wea/54(out19) -> bram53/3
  debus_addrb/54(out19) -> bram53/4
  debus_dinb/54(out19) -> bram53/5
  debus_web/54(out19) -> bram53/6
  debus_addra/55(out18) -> bram54/1
  debus_dina/55(out18) -> bram54/2
  debus_wea/55(out18) -> bram54/3
  debus_addrb/55(out18) -> bram54/4
  debus_dinb/55(out18) -> bram54/5
  debus_web/55(out18) -> bram54/6
  debus_addra/56(out17) -> bram55/1
  debus_dina/56(out17) -> bram55/2
  debus_wea/56(out17) -> bram55/3
  debus_addrb/56(out17) -> bram55/4
  debus_dinb/56(out17) -> bram55/5
  debus_web/56(out17) -> bram55/6
  debus_addra/57(out16) -> bram56/1
  debus_dina/57(out16) -> bram56/2
  debus_wea/57(out16) -> bram56/3
  debus_addrb/57(out16) -> bram56/4
  debus_dinb/57(out16) -> bram56/5
  debus_web/57(out16) -> bram56/6
  debus_addra/58(out15) -> bram57/1
  debus_dina/58(out15) -> bram57/2
  debus_wea/58(out15) -> bram57/3
  debus_addrb/58(out15) -> bram57/4
  debus_dinb/58(out15) -> bram57/5
  debus_web/58(out15) -> bram57/6
  debus_addra/59(out14) -> bram58/1
  debus_dina/59(out14) -> bram58/2
  debus_wea/59(out14) -> bram58/3
  debus_addrb/59(out14) -> bram58/4
  debus_dinb/59(out14) -> bram58/5
  debus_web/59(out14) -> bram58/6
  debus_addra/60(out13) -> bram59/1
  debus_dina/60(out13) -> bram59/2
  debus_wea/60(out13) -> bram59/3
  debus_addrb/60(out13) -> bram59/4
  debus_dinb/60(out13) -> bram59/5
  debus_web/60(out13) -> bram59/6
  debus_addra/61(out12) -> bram60/1
  debus_dina/61(out12) -> bram60/2
  debus_wea/61(out12) -> bram60/3
  debus_addrb/61(out12) -> bram60/4
  debus_dinb/61(out12) -> bram60/5
  debus_web/61(out12) -> bram60/6
  debus_addra/62(out11) -> bram61/1
  debus_dina/62(out11) -> bram61/2
  debus_wea/62(out11) -> bram61/3
  debus_addrb/62(out11) -> bram61/4
  debus_dinb/62(out11) -> bram61/5
  debus_web/62(out11) -> bram61/6
  debus_addra/63(out10) -> bram62/1
  debus_dina/63(out10) -> bram62/2
  debus_wea/63(out10) -> bram62/3
  debus_addrb/63(out10) -> bram62/4
  debus_dinb/63(out10) -> bram62/5
  debus_web/63(out10) -> bram62/6
  debus_addra/64(out9) -> bram63/1
  debus_dina/64(out9) -> bram63/2
  debus_wea/64(out9) -> bram63/3
  debus_addrb/64(out9) -> bram63/4
  debus_dinb/64(out9) -> bram63/5
  debus_web/64(out9) -> bram63/6
  debus_addra/65(out8) -> bram64/1
  debus_dina/65(out8) -> bram64/2
  debus_wea/65(out8) -> bram64/3
  debus_addrb/65(out8) -> bram64/4
  debus_dinb/65(out8) -> bram64/5
  debus_web/65(out8) -> bram64/6
  debus_addra/66(out7) -> bram65/1
  debus_dina/66(out7) -> bram65/2
  debus_wea/66(out7) -> bram65/3
  debus_addrb/66(out7) -> bram65/4
  debus_dinb/66(out7) -> bram65/5
  debus_web/66(out7) -> bram65/6
  debus_addra/67(out6) -> bram66/1
  debus_dina/67(out6) -> bram66/2
  debus_wea/67(out6) -> bram66/3
  debus_addrb/67(out6) -> bram66/4
  debus_dinb/67(out6) -> bram66/5
  debus_web/67(out6) -> bram66/6
  debus_addra/68(out5) -> bram67/1
  debus_dina/68(out5) -> bram67/2
  debus_wea/68(out5) -> bram67/3
  debus_addrb/68(out5) -> bram67/4
  debus_dinb/68(out5) -> bram67/5
  debus_web/68(out5) -> bram67/6
  debus_addra/69(out4) -> bram68/1
  debus_dina/69(out4) -> bram68/2
  debus_wea/69(out4) -> bram68/3
  debus_addrb/69(out4) -> bram68/4
  debus_dinb/69(out4) -> bram68/5
  debus_web/69(out4) -> bram68/6
  debus_addra/70(out3) -> bram69/1
  debus_dina/70(out3) -> bram69/2
  debus_wea/70(out3) -> bram69/3
  debus_addrb/70(out3) -> bram69/4
  debus_dinb/70(out3) -> bram69/5
  debus_web/70(out3) -> bram69/6
  debus_addra/71(out2) -> bram70/1
  debus_dina/71(out2) -> bram70/2
  debus_wea/71(out2) -> bram70/3
  debus_addrb/71(out2) -> bram70/4
  debus_dinb/71(out2) -> bram70/5
  debus_web/71(out2) -> bram70/6
  debus_addra/72(lsb_out1) -> bram71/1
  debus_dina/72(lsb_out1) -> bram71/2
  debus_wea/72(lsb_out1) -> bram71/3
  debus_addrb/72(lsb_out1) -> bram71/4
  debus_dinb/72(lsb_out1) -> bram71/5
  debus_web/72(lsb_out1) -> bram71/6
  bram0/1 -> A_bussify/1(in1)
  bram0/2 -> B_bussify/1(in1)
  bram1/1 -> A_bussify/2(in2)
  bram1/2 -> B_bussify/2(in2)
  bram2/1 -> A_bussify/3(in3)
  bram2/2 -> B_bussify/3(in3)
  bram3/1 -> A_bussify/4(in4)
  bram3/2 -> B_bussify/4(in4)
  bram4/1 -> A_bussify/5(in5)
  bram4/2 -> B_bussify/5(in5)
  bram5/1 -> A_bussify/6(in6)
  bram5/2 -> B_bussify/6(in6)
  bram6/1 -> A_bussify/7(in7)
  bram6/2 -> B_bussify/7(in7)
  bram7/1 -> A_bussify/8(in8)
  bram7/2 -> B_bussify/8(in8)
  bram8/1 -> A_bussify/9(in9)
  bram8/2 -> B_bussify/9(in9)
  bram9/1 -> A_bussify/10(in10)
  bram9/2 -> B_bussify/10(in10)
  bram10/1 -> A_bussify/11(in11)
  bram10/2 -> B_bussify/11(in11)
  bram11/1 -> A_bussify/12(in12)
  bram11/2 -> B_bussify/12(in12)
  bram12/1 -> A_bussify/13(in13)
  bram12/2 -> B_bussify/13(in13)
  bram13/1 -> A_bussify/14(in14)
  bram13/2 -> B_bussify/14(in14)
  bram14/1 -> A_bussify/15(in15)
  bram14/2 -> B_bussify/15(in15)
  bram15/1 -> A_bussify/16(in16)
  bram15/2 -> B_bussify/16(in16)
  bram16/1 -> A_bussify/17(in17)
  bram16/2 -> B_bussify/17(in17)
  bram17/1 -> A_bussify/18(in18)
  bram17/2 -> B_bussify/18(in18)
  bram18/1 -> A_bussify/19(in19)
  bram18/2 -> B_bussify/19(in19)
  bram19/1 -> A_bussify/20(in20)
  bram19/2 -> B_bussify/20(in20)
  bram20/1 -> A_bussify/21(in21)
  bram20/2 -> B_bussify/21(in21)
  bram21/1 -> A_bussify/22(in22)
  bram21/2 -> B_bussify/22(in22)
  bram22/1 -> A_bussify/23(in23)
  bram22/2 -> B_bussify/23(in23)
  bram23/1 -> A_bussify/24(in24)
  bram23/2 -> B_bussify/24(in24)
  bram24/1 -> A_bussify/25(in25)
  bram24/2 -> B_bussify/25(in25)
  bram25/1 -> A_bussify/26(in26)
  bram25/2 -> B_bussify/26(in26)
  bram26/1 -> A_bussify/27(in27)
  bram26/2 -> B_bussify/27(in27)
  bram27/1 -> A_bussify/28(in28)
  bram27/2 -> B_bussify/28(in28)
  bram28/1 -> A_bussify/29(in29)
  bram28/2 -> B_bussify/29(in29)
  bram29/1 -> A_bussify/30(in30)
  bram29/2 -> B_bussify/30(in30)
  bram30/1 -> A_bussify/31(in31)
  bram30/2 -> B_bussify/31(in31)
  bram31/1 -> A_bussify/32(in32)
  bram31/2 -> B_bussify/32(in32)
  bram32/1 -> A_bussify/33(in33)
  bram32/2 -> B_bussify/33(in33)
  bram33/1 -> A_bussify/34(in34)
  bram33/2 -> B_bussify/34(in34)
  bram34/1 -> A_bussify/35(in35)
  bram34/2 -> B_bussify/35(in35)
  bram35/1 -> A_bussify/36(in36)
  bram35/2 -> B_bussify/36(in36)
  bram36/1 -> A_bussify/37(in37)
  bram36/2 -> B_bussify/37(in37)
  bram37/1 -> A_bussify/38(in38)
  bram37/2 -> B_bussify/38(in38)
  bram38/1 -> A_bussify/39(in39)
  bram38/2 -> B_bussify/39(in39)
  bram39/1 -> A_bussify/40(in40)
  bram39/2 -> B_bussify/40(in40)
  bram40/1 -> A_bussify/41(in41)
  bram40/2 -> B_bussify/41(in41)
  bram41/1 -> A_bussify/42(in42)
  bram41/2 -> B_bussify/42(in42)
  bram42/1 -> A_bussify/43(in43)
  bram42/2 -> B_bussify/43(in43)
  bram43/1 -> A_bussify/44(in44)
  bram43/2 -> B_bussify/44(in44)
  bram44/1 -> A_bussify/45(in45)
  bram44/2 -> B_bussify/45(in45)
  bram45/1 -> A_bussify/46(in46)
  bram45/2 -> B_bussify/46(in46)
  bram46/1 -> A_bussify/47(in47)
  bram46/2 -> B_bussify/47(in47)
  bram47/1 -> A_bussify/48(in48)
  bram47/2 -> B_bussify/48(in48)
  bram48/1 -> A_bussify/49(in49)
  bram48/2 -> B_bussify/49(in49)
  bram49/1 -> A_bussify/50(in50)
  bram49/2 -> B_bussify/50(in50)
  bram50/1 -> A_bussify/51(in51)
  bram50/2 -> B_bussify/51(in51)
  bram51/1 -> A_bussify/52(in52)
  bram51/2 -> B_bussify/52(in52)
  bram52/1 -> A_bussify/53(in53)
  bram52/2 -> B_bussify/53(in53)
  bram53/1 -> A_bussify/54(in54)
  bram53/2 -> B_bussify/54(in54)
  bram54/1 -> A_bussify/55(in55)
  bram54/2 -> B_bussify/55(in55)
  bram55/1 -> A_bussify/56(in56)
  bram55/2 -> B_bussify/56(in56)
  bram56/1 -> A_bussify/57(in57)
  bram56/2 -> B_bussify/57(in57)
  bram57/1 -> A_bussify/58(in58)
  bram57/2 -> B_bussify/58(in58)
  bram58/1 -> A_bussify/59(in59)
  bram58/2 -> B_bussify/59(in59)
  bram59/1 -> A_bussify/60(in60)
  bram59/2 -> B_bussify/60(in60)
  bram60/1 -> A_bussify/61(in61)
  bram60/2 -> B_bussify/61(in61)
  bram61/1 -> A_bussify/62(in62)
  bram61/2 -> B_bussify/62(in62)
  bram62/1 -> A_bussify/63(in63)
  bram62/2 -> B_bussify/63(in63)
  bram63/1 -> A_bussify/64(in64)
  bram63/2 -> B_bussify/64(in64)
  bram64/1 -> A_bussify/65(in65)
  bram64/2 -> B_bussify/65(in65)
  bram65/1 -> A_bussify/66(in66)
  bram65/2 -> B_bussify/66(in66)
  bram66/1 -> A_bussify/67(in67)
  bram66/2 -> B_bussify/67(in67)
  bram67/1 -> A_bussify/68(in68)
  bram67/2 -> B_bussify/68(in68)
  bram68/1 -> A_bussify/69(in69)
  bram68/2 -> B_bussify/69(in69)
  bram69/1 -> A_bussify/70(in70)
  bram69/2 -> B_bussify/70(in70)
  bram70/1 -> A_bussify/71(in71)
  bram70/2 -> B_bussify/71(in71)
  bram71/1 -> A_bussify/72(in72)
  bram71/2 -> B_bussify/72(in72)
  A_bussify/1(bus_out) -> A/1
  B_bussify/1(bus_out) -> B/1
